simulink model "Takeoff_Model"  (R2024a)
settings: Solver=VariableStepAuto  StartTime=0.0  StopTime=100  RelTol=1e-3
values from neighbouring files (symbols this model uses):
  deltaE = -10    [run_3DoF_SIM.m]
  gravity = 9.807    [run_3DoF_SIM.m]
  J = 5    [run_3DoF_SIM.m]
  states_init = [0 5000 -0.02056 23.3505 1.0289 0]    [run_3DoF_SIM.m]
  throttle = 0.65    [run_3DoF_SIM.m]
undefined symbols (not defined in the file or in its folder): CD_alpha, CL_alpha, CL_elev, CL_zero, CLEH_alpha, Cm_elev, Cm_zero, Cw, down_wash, M, Sh, Sw, xa, xt
libraries: simulink_extras x4, aerolibatmos2 x1
settings Model: Creator=diego  LastModifiedBy=diego

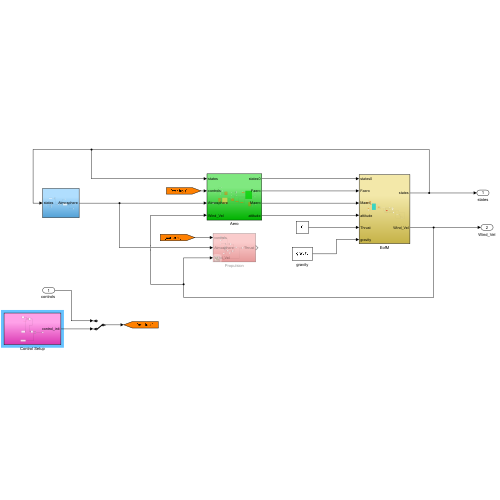
[thumbnail: Simulink's stored preview of the top-level diagram]
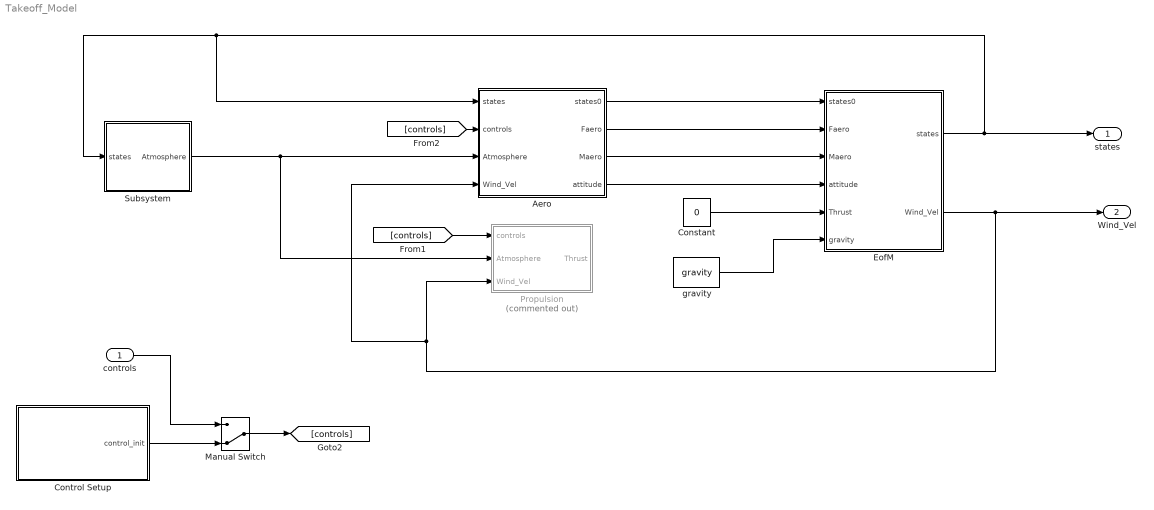
== system Takeoff_Model ==
  "controls " : Inport
  Aero : Subsystem
  Constant : Constant  Value=0
  Control Setup : Subsystem
  EofM : Subsystem
  Manual Switch : ManualSwitch  CurrentSetting=0
  Propulsion : Subsystem  Commented=on
  Subsystem : Subsystem
  gravity : Constant  Value=gravity
  states : Outport
  Wind_Vel : Outport  Port=2
  wires:
  Aero/2(Faero) -> EofM/2(Faero)
  Aero/3(Maero) -> EofM/3(Maero)
  EofM/1(states) -> Subsystem/1(states), Aero/1(states), states/1
  Subsystem/1(Atmosphere) -> Aero/3(Atmosphere), Propulsion/2(Atmosphere)
  EofM/2(Wind_Vel) -> Propulsion/3(Wind_Vel), Aero/4(Wind_Vel), Wind_Vel/1
  Aero/1(states0) -> EofM/1(states0)
  Control Setup/1(control_init) -> Manual Switch/2
  "controls "/1 -> Manual Switch/1
  [controls] -> Aero/2(controls)
  [controls] -> Propulsion/1("controls ")
  Manual Switch/1 -> [controls]
  Aero/4(attitude) -> EofM/4(attitude)
  gravity/1 -> EofM/6(gravity)
  Constant/1 -> EofM/5(Thrust)

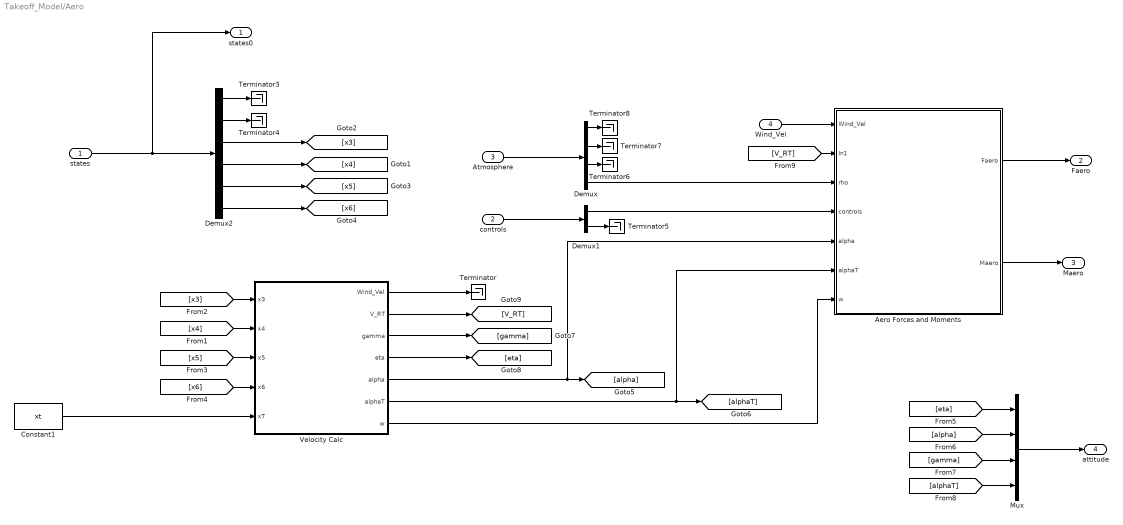
== system Takeoff_Model/Aero ==
  states : Inport
  controls : Inport  Port=2
  Atmosphere : Inport  Port=3
  Wind_Vel : Inport  Port=4
  Aero Forces and Moments : Subsystem
  Constant1 : Constant  Value=xt
  Demux : Demux
  Demux1 : Demux  Outputs=2
  Demux2 : Demux  Outputs=6
  Mux : Mux
  Terminator{,3..8} (7 alike) : Terminator
  Velocity Calc : Subsystem
  states0 : Outport
  Faero : Outport  Port=2
  Maero : Outport  Port=3
  attitude : Outport  Port=4
  wires:
  Atmosphere/1 -> Demux/1
  states/1 -> Demux2/1, states0/1
  Wind_Vel/1 -> Aero Forces and Moments/1(Wind_Vel)
  Demux/4 -> Aero Forces and Moments/3(rho)
  Aero Forces and Moments/1(Faero) -> Faero/1
  Aero Forces and Moments/2(Maero) -> Maero/1
  controls/1 -> Demux1/1
  Demux1/1 -> Aero Forces and Moments/4(controls)
  Constant1/1 -> Velocity Calc/5(xT)
  Velocity Calc/4(eta) -> [eta]
  Velocity Calc/1(Wind_Vel) -> Terminator/1
  Velocity Calc/3(gamma) -> [gamma]
  Demux2/1 -> Terminator3/1
  Demux2/2 -> Terminator4/1
  Demux2/3 -> [x3]
  Demux2/4 -> [x4]
  Demux2/5 -> [x5]
  Demux2/6 -> [x6]
  Demux1/2 -> Terminator5/1
  Demux/1 -> Terminator8/1
  Demux/2 -> Terminator7/1
  Demux/3 -> Terminator6/1
  Velocity Calc/5(alpha) -> Aero Forces and Moments/5(alpha), [alpha]
  Velocity Calc/6(alphaT) -> Aero Forces and Moments/6(alphaT), [alphaT]
  Velocity Calc/7(w) -> Aero Forces and Moments/7(w)
  [x3] -> Velocity Calc/1(x3)
  [x4] -> Velocity Calc/2(x4)
  [x6] -> Velocity Calc/4(x6)
  [x5] -> Velocity Calc/3(x5)
  Mux/1 -> attitude/1
  [eta] -> Mux/1
  [alpha] -> Mux/2
  [gamma] -> Mux/3
  [alphaT] -> Mux/4
  Velocity Calc/2(V_RT) -> [V_RT]
  [V_RT] -> Aero Forces and Moments/2(In1)

== system Takeoff_Model/Control Setup ==
  Add : Sum  Inputs=+++
  Constant : Constant  Value=deltaE
  Constant1 : Constant  Value=throttle
  Degrees to Radians : simulink_extras/Transformations/Degrees to Radians
  Mux : Mux  Inputs=2
  Step : Step  Time=10  After=-15  SampleTime=0
  control_init : Outport
  wires:
  Constant1/1 -> Mux/2
  Degrees to Radians/1 -> Mux/1
  Mux/1 -> control_init/1
  Step/1 -> Add/1
  ? -> Add/2
  Constant/1 -> Add/3
  Add/1 -> Degrees to Radians/1

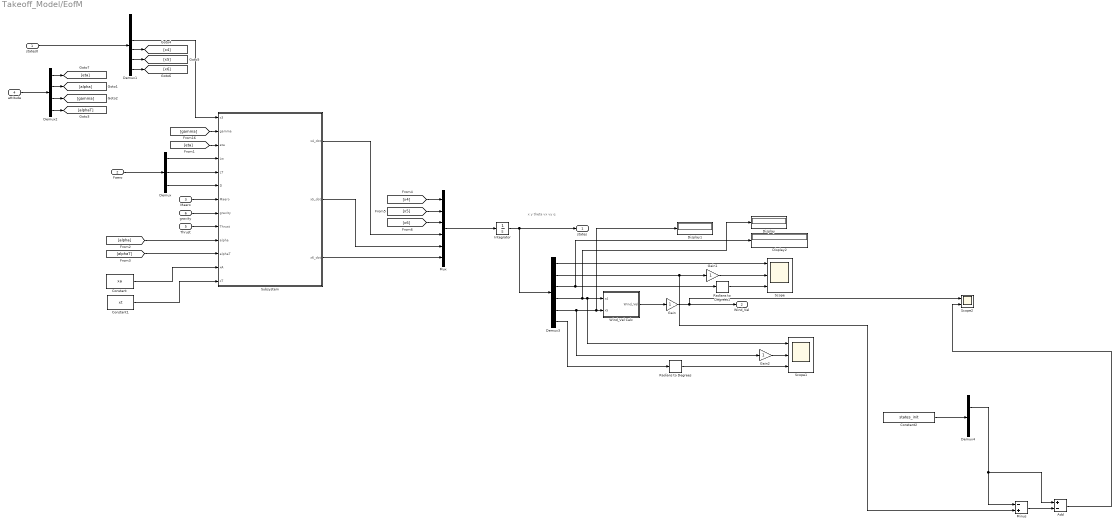
== system Takeoff_Model/EofM ==
  note: x y theta vx vy q
  states0 : Inport
  Faero : Inport  Port=2
  Maero : Inport  Port=3
  attitude : Inport  Port=4
  Thrust : Inport  Port=5
  gravity : Inport  Port=6
  Add : Sum  Inputs=+-
  Constant : Constant  Value=xa
  Constant1 : Constant  Value=xt
  Constant2 : Constant  Value=states_init
  Demux : Demux  Outputs=3
  Demux1 : Demux  Outputs=6
  Demux2 : Demux
  Demux3 : Demux  Outputs=6
  Demux4 : Demux  Outputs=6
  Display : Display
  Display1 : Display
  Display2 : Display
  Gain : Gain
  Gain1 : Gain
  Gain2 : Gain
  Integrator : Integrator  InitialCondition=states_init
  Minus : Sum  Inputs=-+
  Mux : Mux  Inputs=6
  Radians to Degrees : simulink_extras/Transformations/Radians to Degrees
  Radians to Degrees1 : simulink_extras/Transformations/Radians to Degrees
  Scope : Scope  NumInputPorts=3
  Scope1 : Scope  NumInputPorts=3
  Scope2 : Scope  NumInputPorts=2
  Subsystem : Subsystem
  Wind_Vel Calc : Subsystem
  states : Outport
  Wind_Vel : Outport  Port=2
  wires:
  Integrator/1 -> states/1, Demux3/1
  Mux/1 -> Integrator/1
  Faero/1 -> Demux/1
  Demux/1 -> Subsystem/4(Lw)
  Demux/2 -> Subsystem/5(LT)
  Demux/3 -> Subsystem/6(D)
  Maero/1 -> Subsystem/7(Maero)
  gravity/1 -> Subsystem/8(gravity)
  Thrust/1 -> Subsystem/9(Thrust)
  Subsystem/1(x4_dot) -> Mux/4
  Subsystem/2(x5_dot) -> Mux/5
  Subsystem/3(x6_dot) -> Mux/6
  Gain/1 -> Scope2/1, Wind_Vel/1
  attitude/1 -> Demux2/1
  Demux2/1 -> [eta]
  Demux2/2 -> [alpha]
  Demux2/3 -> [gamma]
  Demux2/4 -> [alphaT]
  [eta] -> Subsystem/3(eta)
  [gamma] -> Subsystem/2(gamma)
  [alpha] -> Subsystem/10(alpha)
  [alphaT] -> Subsystem/11(alphaT)
  Demux1/3 -> Subsystem/1(x3)
  Demux1/4 -> [x4]
  Demux1/5 -> [x5]
  Demux1/6 -> [x6]
  [x4] -> Mux/1
  [x5] -> Mux/2
  [x6] -> Mux/3
  Demux3/5 -> Gain2/1, Display1/1, Wind_Vel Calc/2(x5)
  Demux3/4 -> Display/1, Scope1/1, Wind_Vel Calc/1(x4)
  Wind_Vel Calc/1(Wind_Vel) -> Gain/1
  Demux3/1 -> Scope/1
  Demux3/3 -> Display2/1, Radians to Degrees1/1
  Demux3/6 -> Radians to Degrees/1
  states0/1 -> Demux1/1
  Constant/1 -> Subsystem/12("xA ")
  Constant1/1 -> Subsystem/13(xT)
  Radians to Degrees/1 -> Scope1/3
  Radians to Degrees1/1 -> Scope/3
  Gain2/1 -> Scope1/2
  Gain1/1 -> Scope/2
  Constant2/1 -> Demux4/1
  Add/1 -> Scope2/2
  Demux4/2 -> Minus/1, Add/1
  Demux3/2 -> Minus/2, Gain1/1
  Minus/1 -> Add/2

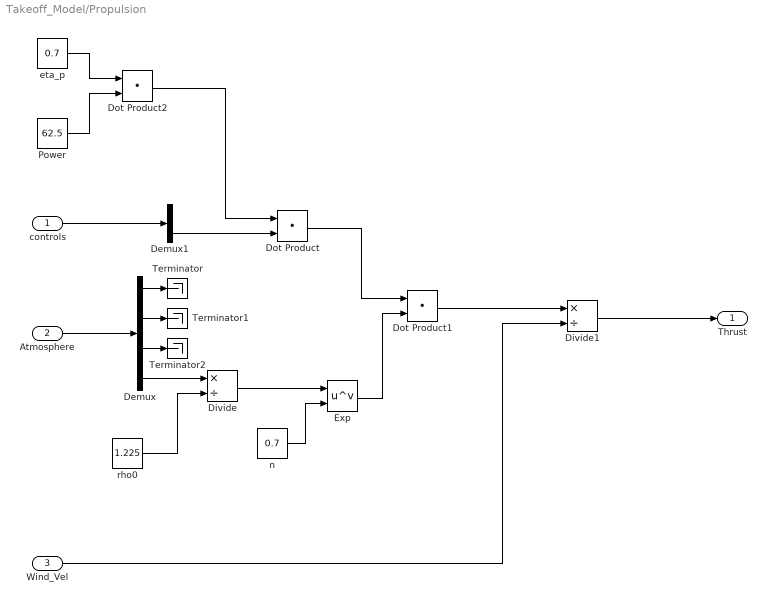
== system Takeoff_Model/Propulsion ==
  "controls " : Inport
  Atmosphere : Inport  Port=2
  Wind_Vel : Inport  Port=3
  Demux : Demux
  Demux1 : Demux  Outputs=2
  Divide : Product  Inputs=*/
  Divide1 : Product  Inputs=*/
  Dot Product : DotProduct  OutDataTypeStr=Inherit: Inherit via internal rule
  Dot Product1 : DotProduct  OutDataTypeStr=Inherit: Inherit via internal rule
  Dot Product2 : DotProduct  OutDataTypeStr=Inherit: Inherit via internal rule
  Exp : Math  Operator=pow
  Power : Constant  Value=62.5
  Terminator : Terminator
  Terminator1 : Terminator
  Terminator2 : Terminator
  eta_p : Constant  Value=0.7
  n : Constant  Value=0.7
  rho0 : Constant  Value=1.225
  Thrust : Outport
  wires:
  "controls "/1 -> Demux1/1
  Atmosphere/1 -> Demux/1
  Demux/4 -> Divide/1
  rho0/1 -> Divide/2
  Divide/1 -> Exp/1
  n/1 -> Exp/2
  Dot Product/1 -> Dot Product1/1
  Exp/1 -> Dot Product1/2
  Divide1/1 -> Thrust/1
  Wind_Vel/1 -> Divide1/2
  Dot Product1/1 -> Divide1/1
  Dot Product2/1 -> Dot Product/1
  Power/1 -> Dot Product2/2
  eta_p/1 -> Dot Product2/1
  Demux1/2 -> Dot Product/2
  Demux/1 -> Terminator/1
  Demux/2 -> Terminator1/1
  Demux/3 -> Terminator2/1

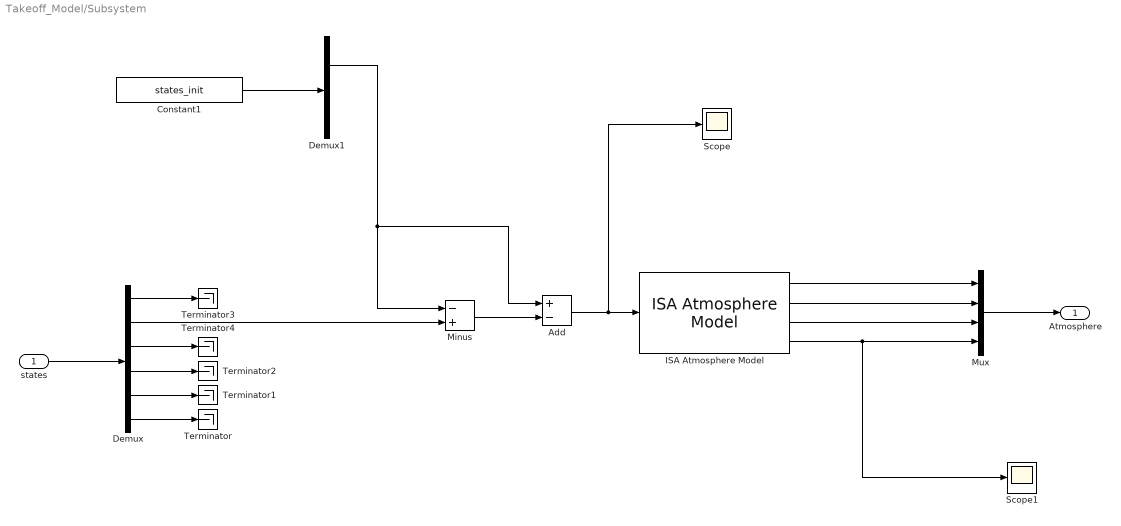
== system Takeoff_Model/Subsystem ==
  states : Inport
  Add : Sum  Inputs=+-
  Constant1 : Constant  Value=states_init
  Demux : Demux  Outputs=6
  Demux1 : Demux  Outputs=6
  ISA Atmosphere Model : aerolibatmos2/ISA Atmosphere Model  useExtended=off  action=Warning  custom=off  viscosityOut=off  g=9.80665  gamma=1.4  R=287.0531  L=0.0065  h_trop=11000  h_strat=20000  rho0=1.225  P0=101325  T0=288.15  h0=0  S=110.4  Tref=273.15  muref=1.716e-5
  Minus : Sum  Inputs=-+
  Mux : Mux
  Scope : Scope
  Scope1 : Scope
  Terminator{,1..4} (5 alike) : Terminator
  Atmosphere : Outport
  wires:
  ISA Atmosphere Model/1 -> Mux/1
  ISA Atmosphere Model/2 -> Mux/2
  ISA Atmosphere Model/3 -> Mux/3
  Mux/1 -> Atmosphere/1
  states/1 -> Demux/1
  Demux/6 -> Terminator/1
  Demux/5 -> Terminator1/1
  Demux/4 -> Terminator2/1
  Demux/1 -> Terminator3/1
  Demux/3 -> Terminator4/1
  Constant1/1 -> Demux1/1
  Demux1/2 -> Minus/1, Add/1
  Demux/2 -> Minus/2
  Minus/1 -> Add/2
  Add/1 -> Scope/1, ISA Atmosphere Model/1
  ISA Atmosphere Model/4 -> Scope1/1, Mux/4

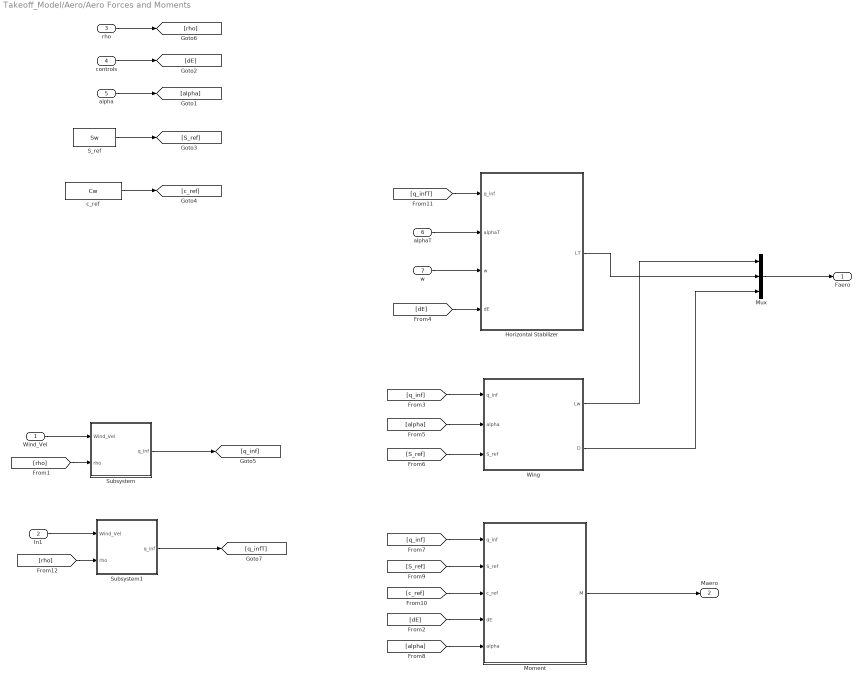
== system Takeoff_Model/Aero/Aero Forces and Moments ==
  Wind_Vel : Inport
  In1 : Inport  Port=2
  rho : Inport  Port=3
  controls : Inport  Port=4
  alpha : Inport  Port=5
  alphaT : Inport  Port=6
  w : Inport  Port=7
  Horizontal Stabilizer : Subsystem
  Moment : Subsystem
  Mux : Mux  Inputs=3
  S_ref : Constant  Value=Sw
  Subsystem : Subsystem
  Subsystem1 : Subsystem
  Wing : Subsystem
  c_ref : Constant  Value=Cw
  Faero : Outport
  Maero : Outport  Port=2
  wires:
  Mux/1 -> Faero/1
  Wind_Vel/1 -> Subsystem/1(Wind_Vel)
  Horizontal Stabilizer/1(LT) -> Mux/2
  Wing/1(Lw) -> Mux/1
  Wing/2(D) -> Mux/3
  Moment/1(M) -> Maero/1
  w/1 -> Horizontal Stabilizer/3(w)
  alphaT/1 -> Horizontal Stabilizer/2(alphaT)
  controls/1 -> [dE]
  [dE] -> Horizontal Stabilizer/4(dE)
  c_ref/1 -> [c_ref]
  S_ref/1 -> [S_ref]
  alpha/1 -> [alpha]
  Subsystem/1(q_inf) -> [q_inf]
  [q_infT] -> Horizontal Stabilizer/1(q_inf)
  [dE] -> Moment/4(dE)
  [q_inf] -> Wing/1(q_inf)
  [alpha] -> Wing/2(alpha)
  [S_ref] -> Wing/3(S_ref)
  [c_ref] -> Moment/3(c_ref)
  [S_ref] -> Moment/2(S_ref)
  [alpha] -> Moment/5(alpha)
  [q_inf] -> Moment/1(q_inf)
  rho/1 -> [rho]
  [rho] -> Subsystem/2(rho)
  [rho] -> Subsystem1/2(rho)
  Subsystem1/1(q_inf) -> [q_infT]
  In1/1 -> Subsystem1/1(Wind_Vel)

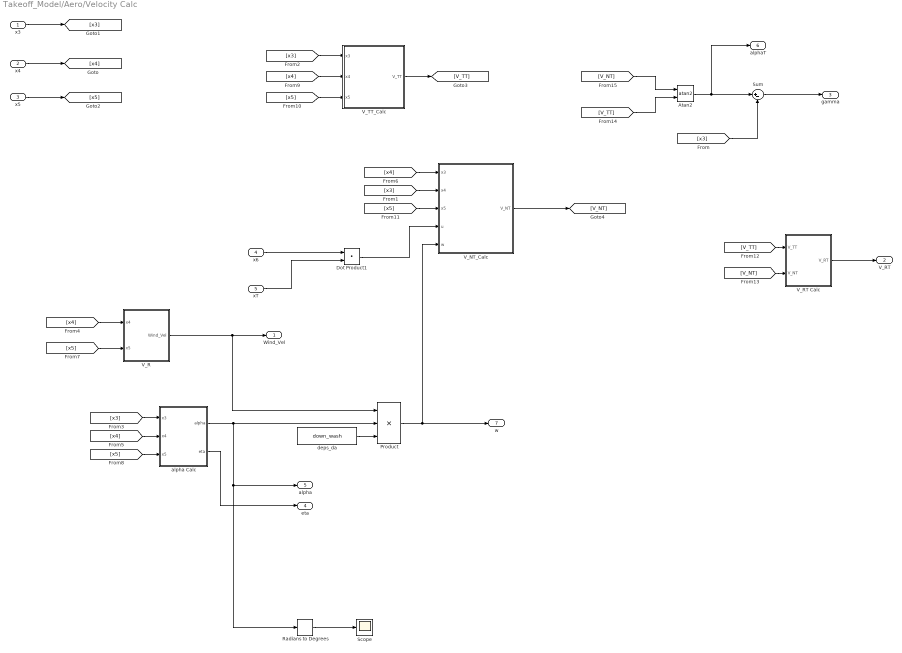
== system Takeoff_Model/Aero/Velocity Calc ==
  x3 : Inport
  x4 : Inport  Port=2
  x5 : Inport  Port=3
  x6 : Inport  Port=4
  xT : Inport  Port=5
  Atan2 : Trigonometry  Operator=atan2
  Dot Product1 : DotProduct  OutDataTypeStr=Inherit: Inherit via internal rule
  Product : Product  Inputs=3
  Radians to Degrees : simulink_extras/Transformations/Radians to Degrees
  Scope : Scope
  Sum : Sum  Inputs=|+-
  V_NT_Calc : Subsystem
  V_R : Subsystem
  V_RT Calc : Subsystem
  V_TT_Calc : Subsystem
  alpha Calc : Subsystem
  deps_da : Constant  Value=down_wash
  Wind_Vel : Outport
  V_RT : Outport  Port=2
  gamma : Outport  Port=3
  eta : Outport  Port=4
  alpha : Outport  Port=5
  alphaT : Outport  Port=6
  w : Outport  Port=7
  wires:
  V_R/1(Wind_Vel) -> Product/1, Wind_Vel/1
  x5/1 -> [x5]
  x4/1 -> [x4]
  x6/1 -> Dot Product1/1
  deps_da/1 -> Product/3
  Dot Product1/1 -> V_NT_Calc/4(u)
  Product/1 -> V_NT_Calc/5(w), w/1
  x3/1 -> [x3]
  Atan2/1 -> alphaT/1, Sum/1
  Sum/1 -> gamma/1
  alpha Calc/2(eta) -> eta/1
  xT/1 -> Dot Product1/2
  [x3] -> Sum/2
  [x3] -> V_NT_Calc/2(x4)
  [x3] -> V_TT_Calc/1(x3)
  [x3] -> alpha Calc/1(x3)
  [x4] -> V_R/1(x4)
  [x4] -> alpha Calc/2(x4)
  [x4] -> V_NT_Calc/1(x3)
  [x5] -> V_R/2(x5)
  [x5] -> alpha Calc/3(x5)
  [x4] -> V_TT_Calc/2(x4)
  V_TT_Calc/1(V_TT) -> [V_TT]
  V_NT_Calc/1(V_NT) -> [V_NT]
  [V_TT] -> V_RT Calc/1(V_TT)
  [V_NT] -> V_RT Calc/2(V_NT)
  [V_NT] -> Atan2/1
  [V_TT] -> Atan2/2
  V_RT Calc/1(V_RT) -> V_RT/1
  [x5] -> V_TT_Calc/3(x5)
  [x5] -> V_NT_Calc/3(x5)
  alpha Calc/1(alpha) -> Product/2, Radians to Degrees/1, alpha/1
  Radians to Degrees/1 -> Scope/1

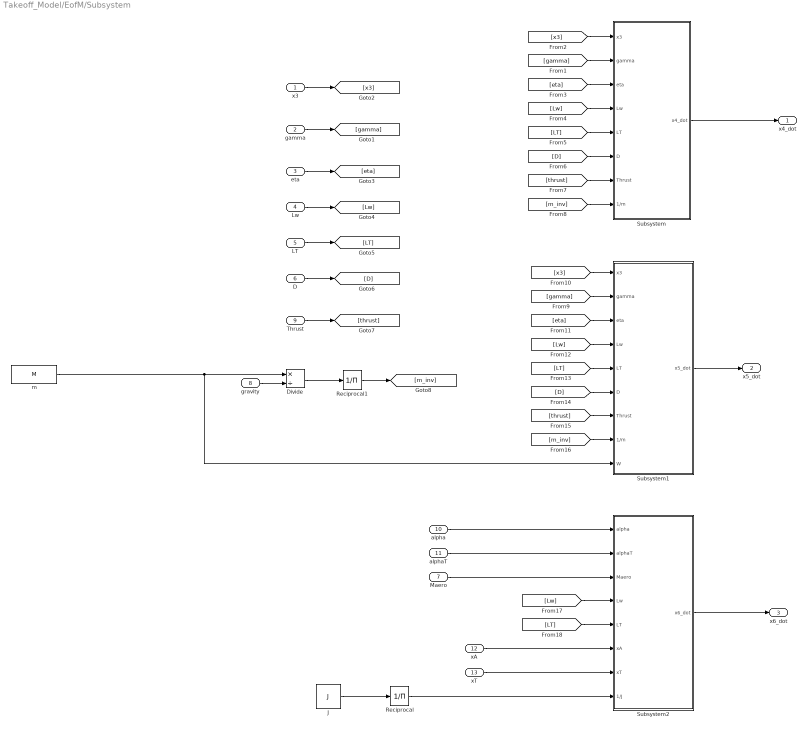
== system Takeoff_Model/EofM/Subsystem ==
  x3 : Inport
  gamma : Inport  Port=2
  eta : Inport  Port=3
  Lw : Inport  Port=4
  LT : Inport  Port=5
  D : Inport  Port=6
  Maero : Inport  Port=7
  gravity : Inport  Port=8
  Thrust : Inport  Port=9
  alpha : Inport  Port=10
  alphaT : Inport  Port=11
  "xA " : Inport  Port=12
  xT : Inport  Port=13
  Divide : Product  Inputs=*/
  J : Constant  Value=J
  Reciprocal : Product  Inputs=/
  Reciprocal1 : Product  Inputs=/
  Subsystem : Subsystem
  Subsystem1 : Subsystem
  Subsystem2 : Subsystem
  m : Constant  Value=M
  x4_dot : Outport
  x5_dot : Outport  Port=2
  x6_dot : Outport  Port=3
  wires:
  Reciprocal/1 -> Subsystem2/8(1/J)
  J/1 -> Reciprocal/1
  Thrust/1 -> [thrust]
  Reciprocal1/1 -> [m_inv]
  Subsystem/1(x4_dot) -> x4_dot/1
  Subsystem1/1(x5_dot) -> x5_dot/1
  alpha/1 -> Subsystem2/1(alpha)
  alphaT/1 -> Subsystem2/2(alphaT)
  Maero/1 -> Subsystem2/3(Maero)
  "xA "/1 -> Subsystem2/6(xA)
  xT/1 -> Subsystem2/7(xT)
  Subsystem2/1(x6_dot) -> x6_dot/1
  x3/1 -> [x3]
  gamma/1 -> [gamma]
  eta/1 -> [eta]
  Lw/1 -> [Lw]
  D/1 -> [D]
  LT/1 -> [LT]
  [x3] -> Subsystem/1(x3)
  [gamma] -> Subsystem/2(gamma)
  [m_inv] -> Subsystem/8(1/m)
  [thrust] -> Subsystem/7(Thrust)
  [D] -> Subsystem/6(D)
  [LT] -> Subsystem/5(LT)
  [Lw] -> Subsystem/4(Lw)
  [eta] -> Subsystem/3(eta)
  [x3] -> Subsystem1/1(x3)
  [D] -> Subsystem1/6(D)
  [thrust] -> Subsystem1/7(Thrust)
  [Lw] -> Subsystem1/4(Lw)
  [gamma] -> Subsystem1/2(gamma)
  [eta] -> Subsystem1/3(eta)
  [m_inv] -> Subsystem1/8(1/m)
  [LT] -> Subsystem1/5(LT)
  m/1 -> Divide/1, Subsystem1/9(W)
  [Lw] -> Subsystem2/4(Lw)
  [LT] -> Subsystem2/5(LT)
  Divide/1 -> Reciprocal1/1
  gravity/1 -> Divide/2

== system Takeoff_Model/EofM/Wind_Vel Calc ==
  x4 : Inport
  x5 : Inport  Port=2
  Sqrt : Sqrt
  Square : Math  Operator=square
  Square1 : Math  Operator=square
  Sum : Sum  Inputs=|++
  Wind_Vel : Outport
  wires:
  Sqrt/1 -> Wind_Vel/1
  x5/1 -> Square1/1
  Square1/1 -> Sum/2
  Sum/1 -> Sqrt/1
  x4/1 -> Square/1
  Square/1 -> Sum/1

== system Takeoff_Model/Aero/Aero Forces and Moments/Horizontal Stabilizer ==
  q_inf : Inport
  alphaT : Inport  Port=2
  w : Inport  Port=3
  dE : Inport  Port=4
  " " : DotProduct  OutDataTypeStr=Inherit: Inherit via internal rule
  Add : Sum
  Constant1 : Constant  Value=CLEH_alpha
  Constant2 : Constant  Value=CL_elev
  Dot Product : DotProduct  OutDataTypeStr=Inherit: Inherit via internal rule
  Dot Product1 : DotProduct  OutDataTypeStr=Inherit: Inherit via internal rule
  Dot Product2 : DotProduct  OutDataTypeStr=Inherit: Inherit via internal rule
  Sh : Constant  Value=Sh
  Sum : Sum  Inputs=|++
  LT : Outport
  wires:
  Sh/1 -> " "/2
  " "/1 -> LT/1
  Constant2/1 -> Dot Product/2
  dE/1 -> Dot Product/1
  alphaT/1 -> Add/1
  w/1 -> Add/2
  Constant1/1 -> Dot Product1/1
  Add/1 -> Dot Product1/2
  Dot Product1/1 -> Sum/2
  Dot Product/1 -> Sum/1
  q_inf/1 -> Dot Product2/1
  Sum/1 -> Dot Product2/2
  Dot Product2/1 -> " "/1

== system Takeoff_Model/Aero/Aero Forces and Moments/Moment ==
  q_inf : Inport
  S_ref : Inport  Port=2
  c_ref : Inport  Port=3
  dE : Inport  Port=4
  alpha : Inport  Port=5
  1-D Lookup Table : Lookup_n-D  NumberOfTableDimensions=1  BreakpointsForDimension1=Cm_elev(:, 1)  Table=Cm_elev(:, 2)  InternalRulePriority=Speed  RndMeth=Simplest
  Add : Sum
  CM0 : Constant  Value=Cm_zero
  Dot Product{1..3,6} (4 alike) : DotProduct  OutDataTypeStr=Inherit: Inherit via internal rule
  M : Outport
  wires:
  Dot Product1/1 -> Dot Product2/1
  q_inf/1 -> Dot Product1/1
  c_ref/1 -> Dot Product6/2
  S_ref/1 -> Dot Product2/2
  Dot Product6/1 -> M/1
  Dot Product2/1 -> Dot Product6/1
  dE/1 -> Dot Product3/2
  alpha/1 -> 1-D Lookup Table/1
  1-D Lookup Table/1 -> Dot Product3/1
  CM0/1 -> Add/1
  Dot Product3/1 -> Add/2
  Add/1 -> Dot Product1/2

== system Takeoff_Model/Aero/Aero Forces and Moments/Subsystem ==
  Wind_Vel : Inport
  rho : Inport  Port=2
  Constant : Constant  Value=0.5
  Product : Product  Inputs=3
  Square : Math  Operator=square
  q_inf : Outport
  wires:
  Wind_Vel/1 -> Square/1
  Square/1 -> Product/1
  rho/1 -> Product/2
  Constant/1 -> Product/3
  Product/1 -> q_inf/1

== system Takeoff_Model/Aero/Aero Forces and Moments/Subsystem1 ==
  Wind_Vel : Inport
  rho : Inport  Port=2
  Constant : Constant  Value=0.5
  Product : Product  Inputs=3
  Square : Math  Operator=square
  q_inf : Outport
  wires:
  Wind_Vel/1 -> Square/1
  Square/1 -> Product/1
  rho/1 -> Product/2
  Constant/1 -> Product/3
  Product/1 -> q_inf/1

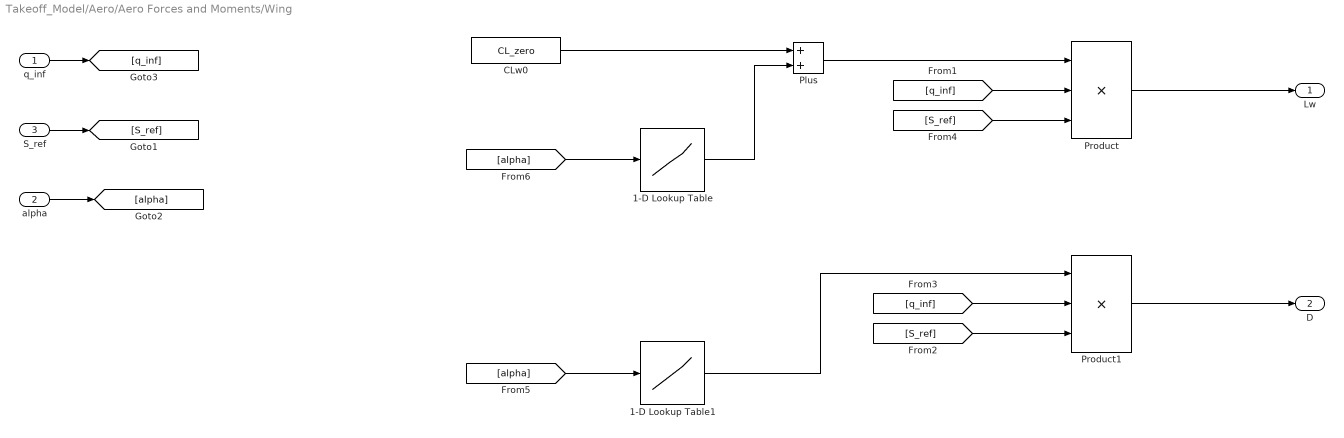
== system Takeoff_Model/Aero/Aero Forces and Moments/Wing ==
  q_inf : Inport
  alpha : Inport  Port=2
  S_ref : Inport  Port=3
  1-D Lookup Table : Lookup_n-D  NumberOfTableDimensions=1  BreakpointsForDimension1=CL_alpha(:, 1)  Table=CL_alpha(:, 2)  InternalRulePriority=Speed  RndMeth=Simplest
  1-D Lookup Table1 : Lookup_n-D  NumberOfTableDimensions=1  BreakpointsForDimension1=CD_alpha(:, 1)  Table=CD_alpha(:, 2)  InternalRulePriority=Speed  RndMeth=Simplest
  CLw0 : Constant  Value=CL_zero
  Plus : Sum
  Product : Product  Inputs=3
  Product1 : Product  Inputs=3
  Lw : Outport
  D : Outport  Port=2
  wires:
  Product/1 -> Lw/1
  CLw0/1 -> Plus/1
  Plus/1 -> Product/1
  q_inf/1 -> [q_inf]
  S_ref/1 -> [S_ref]
  [S_ref] -> Product/3
  1-D Lookup Table/1 -> Plus/2
  alpha/1 -> [alpha]
  [alpha] -> 1-D Lookup Table1/1
  [alpha] -> 1-D Lookup Table/1
  [q_inf] -> Product/2
  Product1/1 -> D/1
  [S_ref] -> Product1/3
  [q_inf] -> Product1/2
  1-D Lookup Table1/1 -> Product1/1

== system Takeoff_Model/Aero/Velocity Calc/V_NT_Calc ==
  x3 : Inport
  x4 : Inport  Port=2
  x5 : Inport  Port=3
  u : Inport  Port=4
  w : Inport  Port=5
  Cos : Trigonometry
  Dot Product : DotProduct  OutDataTypeStr=Inherit: Inherit via internal rule
  Dot Product1 : DotProduct  OutDataTypeStr=Inherit: Inherit via internal rule
  Sin : Trigonometry  Operator=cos
  Subtract : Sum  Inputs=+-
  Sum2 : Sum  Inputs=|++
  Sum3 : Sum  Inputs=|+-
  V_NT : Outport
  wires:
  u/1 -> Sum2/2
  w/1 -> Sum3/2
  Sum2/1 -> Sum3/1
  Sum3/1 -> V_NT/1
  x4/1 -> Dot Product/2
  Dot Product/1 -> Subtract/1
  x5/1 -> Dot Product1/2
  x3/1 -> Sin/1, Cos/1
  Dot Product1/1 -> Subtract/2
  Sin/1 -> Dot Product1/1
  Cos/1 -> Dot Product/1
  Subtract/1 -> Sum2/1

== system Takeoff_Model/Aero/Velocity Calc/V_R ==
  x4 : Inport
  x5 : Inport  Port=2
  Sqrt : Sqrt
  Square : Math  Operator=square
  Square1 : Math  Operator=square
  Sum : Sum  Inputs=|++
  Wind_Vel : Outport
  wires:
  Sqrt/1 -> Wind_Vel/1
  x5/1 -> Square1/1
  Square1/1 -> Sum/2
  Sum/1 -> Sqrt/1
  x4/1 -> Square/1
  Square/1 -> Sum/1

== system Takeoff_Model/Aero/Velocity Calc/V_RT Calc ==
  V_TT : Inport
  V_NT : Inport  Port=2
  Sqrt : Sqrt
  Square : Math  Operator=square
  Square1 : Math  Operator=square
  Sum : Sum  Inputs=|++
  V_RT : Outport
  wires:
  V_TT/1 -> Square/1
  Sqrt/1 -> V_RT/1
  Square/1 -> Sum/1
  Sum/1 -> Sqrt/1
  V_NT/1 -> Square1/1
  Square1/1 -> Sum/2

== system Takeoff_Model/Aero/Velocity Calc/V_TT_Calc ==
  x3 : Inport
  x4 : Inport  Port=2
  x5 : Inport  Port=3
  Cos : Trigonometry  Operator=cos
  Dot Product : DotProduct  OutDataTypeStr=Inherit: Inherit via internal rule
  Dot Product1 : DotProduct  OutDataTypeStr=Inherit: Inherit via internal rule
  Sin : Trigonometry
  Subtract : Sum  Inputs=+-
  V_TT : Outport
  wires:
  Subtract/1 -> V_TT/1
  x3/1 -> Sin/1, Cos/1
  Cos/1 -> Dot Product/1
  x4/1 -> Dot Product/2
  Sin/1 -> Dot Product1/1
  x5/1 -> Dot Product1/2
  Dot Product/1 -> Subtract/1
  Dot Product1/1 -> Subtract/2

== system Takeoff_Model/Aero/Velocity Calc/alpha Calc ==
  x3 : Inport
  x4 : Inport  Port=2
  x5 : Inport  Port=3
  Atan2 : Trigonometry  Operator=atan2
  Sum : Sum  Inputs=|++
  alpha : Outport
  eta : Outport  Port=2
  wires:
  x3/1 -> Sum/2
  Atan2/1 -> Sum/1, eta/1
  x5/1 -> Atan2/1
  x4/1 -> Atan2/2
  Sum/1 -> alpha/1

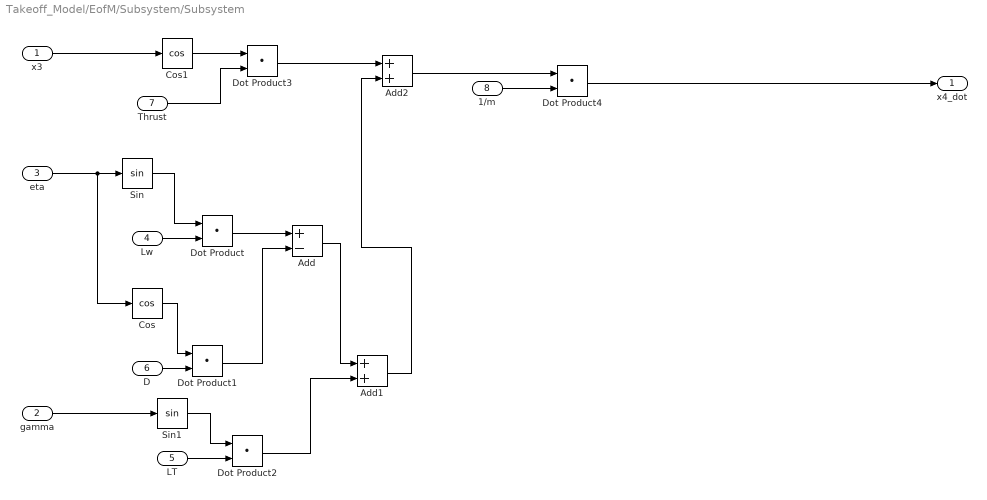
== system Takeoff_Model/EofM/Subsystem/Subsystem ==
  x3 : Inport
  gamma : Inport  Port=2
  eta : Inport  Port=3
  Lw : Inport  Port=4
  LT : Inport  Port=5
  D : Inport  Port=6
  Thrust : Inport  Port=7
  1/m : Inport  Port=8
  Add : Sum  Inputs=+-
  Add1 : Sum
  Add2 : Sum
  Cos : Trigonometry  Operator=cos
  Cos1 : Trigonometry  Operator=cos
  Dot Product{,1..4} (5 alike) : DotProduct  OutDataTypeStr=Inherit: Inherit via internal rule
  Sin : Trigonometry
  Sin1 : Trigonometry
  x4_dot : Outport
  wires:
  Add2/1 -> Dot Product4/1
  Cos/1 -> Dot Product1/1
  Add/1 -> Add1/1
  Sin/1 -> Dot Product/1
  Dot Product2/1 -> Add1/2
  LT/1 -> Dot Product2/2
  Dot Product3/1 -> Add2/1
  Dot Product1/1 -> Add/2
  eta/1 -> Cos/1, Sin/1
  Cos1/1 -> Dot Product3/1
  1/m/1 -> Dot Product4/2
  Sin1/1 -> Dot Product2/1
  Dot Product/1 -> Add/1
  Add1/1 -> Add2/2
  gamma/1 -> Sin1/1
  D/1 -> Dot Product1/2
  x3/1 -> Cos1/1
  Lw/1 -> Dot Product/2
  Thrust/1 -> Dot Product3/2
  Dot Product4/1 -> x4_dot/1

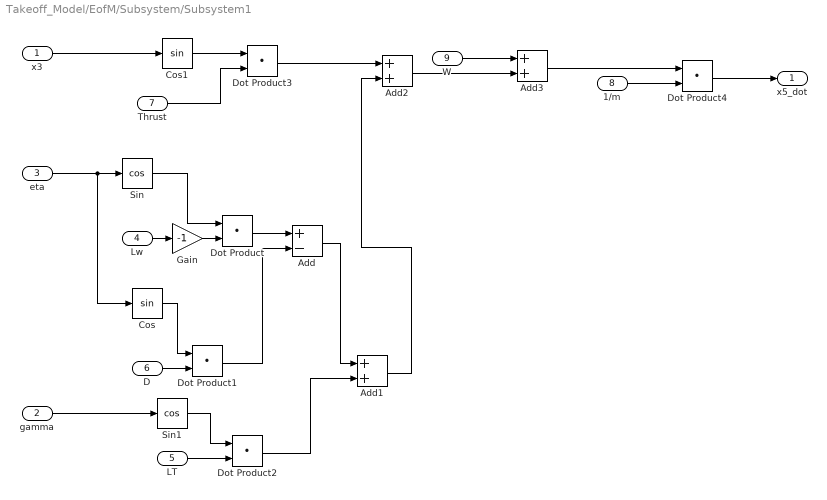
== system Takeoff_Model/EofM/Subsystem/Subsystem1 ==
  x3 : Inport
  gamma : Inport  Port=2
  eta : Inport  Port=3
  Lw : Inport  Port=4
  LT : Inport  Port=5
  D : Inport  Port=6
  Thrust : Inport  Port=7
  1/m : Inport  Port=8
  W : Inport  Port=9
  Add : Sum  Inputs=+-
  Add1 : Sum
  Add2 : Sum
  Add3 : Sum
  Cos : Trigonometry
  Cos1 : Trigonometry
  Dot Product{,1..4} (5 alike) : DotProduct  OutDataTypeStr=Inherit: Inherit via internal rule
  Gain : Gain  Gain=-1
  Sin : Trigonometry  Operator=cos
  Sin1 : Trigonometry  Operator=cos
  x5_dot : Outport
  wires:
  Dot Product2/1 -> Add1/2
  Add1/1 -> Add2/2
  Sin1/1 -> Dot Product2/1
  Cos1/1 -> Dot Product3/1
  Dot Product/1 -> Add/1
  Add2/1 -> Add3/2
  Cos/1 -> Dot Product1/1
  Sin/1 -> Dot Product/1
  Add/1 -> Add1/1
  Dot Product3/1 -> Add2/1
  Lw/1 -> Gain/1
  1/m/1 -> Dot Product4/2
  Dot Product4/1 -> x5_dot/1
  LT/1 -> Dot Product2/2
  D/1 -> Dot Product1/2
  Dot Product1/1 -> Add/2
  eta/1 -> Cos/1, Sin/1
  gamma/1 -> Sin1/1
  Thrust/1 -> Dot Product3/2
  x3/1 -> Cos1/1
  Gain/1 -> Dot Product/2
  W/1 -> Add3/1
  Add3/1 -> Dot Product4/1

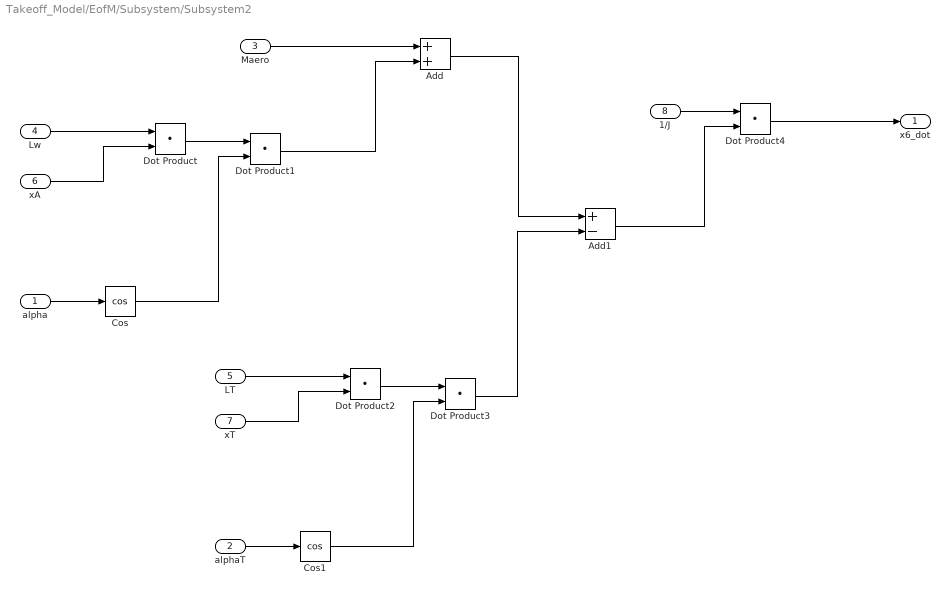
== system Takeoff_Model/EofM/Subsystem/Subsystem2 ==
  alpha : Inport
  alphaT : Inport  Port=2
  Maero : Inport  Port=3
  Lw : Inport  Port=4
  LT : Inport  Port=5
  xA : Inport  Port=6
  xT : Inport  Port=7
  1/J : Inport  Port=8
  Add : Sum
  Add1 : Sum  Inputs=+-
  Cos : Trigonometry  Operator=cos
  Cos1 : Trigonometry  Operator=cos
  Dot Product{,1..4} (5 alike) : DotProduct  OutDataTypeStr=Inherit: Inherit via internal rule
  x6_dot : Outport
  wires:
  Maero/1 -> Add/1
  Lw/1 -> Dot Product/1
  xA/1 -> Dot Product/2
  alpha/1 -> Cos/1
  Dot Product/1 -> Dot Product1/1
  Cos/1 -> Dot Product1/2
  Dot Product1/1 -> Add/2
  xT/1 -> Dot Product2/2
  Cos1/1 -> Dot Product3/2
  LT/1 -> Dot Product2/1
  Dot Product2/1 -> Dot Product3/1
  alphaT/1 -> Cos1/1
  Add/1 -> Add1/1
  Dot Product3/1 -> Add1/2
  1/J/1 -> Dot Product4/1
  Add1/1 -> Dot Product4/2
  Dot Product4/1 -> x6_dot/1
